simulink model "lift_design"  (R2020b)
settings: Solver=VariableStepAuto  StartTime=0.0  StopTime=10.0  RelTol=1e-3
undefined symbols (not defined in the file): sigbuilder_block
settings Model: EnablePacing=on  PacingRate=0.400000  Creator=shivanshu shukla  LastModifiedBy=shivanshu shukla

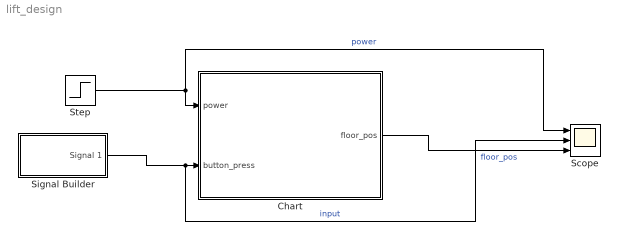
== system lift_design ==
  Chart : Stateflow chart  TreatAsAtomicUnit=on
  Scope : Scope  NumInputPorts=3
  Signal Builder : Subsystem  Tag=STV Subsys  LoadFcn=sigbuilder_block('load');  StartFcn=sigbuilder_block('start');  StopFcn=sigbuilder_block('stop');  ClipboardFcn=sigbuilder_block('clipboard');  mask(Sigbuilder block){tuvar=[0:10]}
      mask help: Simulink:masks:SigbuilderBlock_MD
      mask init:
      | if ~strcmp(get_param(bdroot(gcbh),'SimulationStatus'),'stopped') tuvar = sigbuilder_block('maskInit'); end
      settings: CopyFcn=sigbuilder_block('copy');  DeleteFcn=sigbuilder_block('delete');  ModelCloseFcn=sigbuilder_block('modelClose');  PreSaveFcn=sigbuilder_block('preSave');  PauseFcn=sigbuilder_block('pause');  ContinueFcn=sigbuilder_block('continue');  NameChangeFcn=sigbuilder_block('namechange');  OpenFcn=sigbuilder_block('open',[437.6 153 550.4 359.25 ]);  CloseFcn=sigbuilder_block('close');
      mask Display: plot(0, 0, 100, 100,[2, 2, 32, 32, 2], [68, 8, 8, 68, 68],[32, 2], [38, 38], [32, 19, 2],[53, 60, 44], [32, 17, 17, 2],[16, 16, 31, 31]);txt = getActiveGroup(gcbh);text(2, 100, txt,'verticalAlignment', 'top');
  Step : Step  Time=2  SampleTime=0
  wires:
  Step/1 -> Chart/1(power), Scope/1  "power"
  Signal Builder/1(Signal 1) -> Scope/2, Chart/2(button_press)  "input"
  Chart/1(floor_pos) -> Scope/3  "floor_pos"

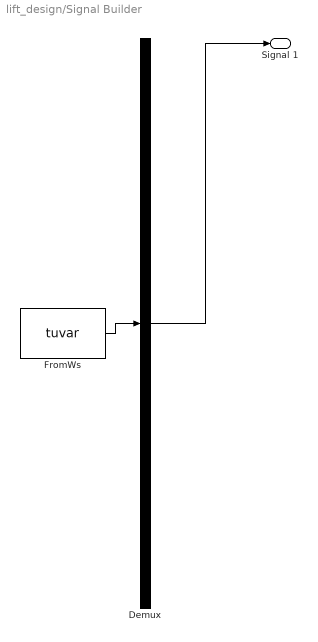
== system lift_design/Signal Builder ==
  Demux : Demux  Tag=STV Demux  Outputs=1
      settings: DisplayOption=none
  FromWs : FromWorkspace  Tag=STV FromWs  VariableName=tuvar
      SigBuilderData=|
      | common.afterFinalStr = 'Extrapolate'
      | common.sampleTime = 0
      | dataSet.timeRange = [0 10]
      | dataSet.name = 'Group 1'
      | sbobj.Groups.Name = 'Group 1'
      | sbobj.Groups.Signals.Name = 'Signal 1'
      | sbobj.Groups.Signals.XData = [0 3 3 4 4 6 6 7 7 10]
      | sbobj.Groups.Signals.YData = [0 0 2 2 5 5.05 3 3 0 0.05]
  Signal 1 : Outport  Tag=STV Outport
  wires:
  Demux/1 -> Signal 1/1
  FromWs/1 -> Demux/1

== stateflow chart lift_design/Chart ==
  settings: executeAtInitialization=1
  state PowerOff
  state PowerOn
    state Lift_moment_to_floor
      state floor2
      state floor5
      state floor3
      state floor4
      state floor1
        entry:
        floor_pos=1;
      (default) -> floor1
      floor4 -> floor5 [order 1] : [button_press>4]{floor_pos=floor_pos+1;}
      floor2 -> floor3 [order 1] : [button_press>2]{floor_pos=floor_pos+1;}
      floor1 -> floor2 : [button_press>1]{floor_pos=floor_pos+1;}
      floor3 -> floor4 [order 1] : [button_press>3]{floor_pos=floor_pos+1;}
      floor2 -> floor1 [order 2] : [button_press<2]{floor_pos=floor_pos-1;}
      floor3 -> floor2 [order 2] : [button_press<3]{floor_pos=floor_pos-1;}
      floor5 -> floor4 : [button_press<5]{floor_pos=floor_pos-1;}
      floor4 -> floor3 [order 2] : [button_press<4]{floor_pos=floor_pos-1;}
    state FAN_Mode [commented out]
      state FanOff [commented out]
        en:
        fan=0;
      state FanOn [commented out]
        en:
        fan=1;
      (default) -> FanOff [commented out]
      FanOff -> FanOn [commented out] : [m==1]
      FanOn -> FanOff [commented out] : [m==0]
    (default) -> Lift_moment_to_floor
  (default) -> PowerOff
  PowerOff -> PowerOn : [power==1]
  PowerOn -> PowerOff : [power==0]
  data: power input; floor_pos output; button_press input
